simulink model "Control_Of_SinglePhaseACMotor"  (R2024b)
settings: Solver=FixedStepDiscrete  StartTime=0.0  StopTime=10.0  FixedStep=50e-6  RelTol=1e-3
undefined symbols (not defined in the file): DiscIntNeverNeededParam, Frequency
libraries: simulink x1
settings Model: DataDictionary=Control_Of_SinglePhaseACMotor.sldd  Creator=User  LastModifiedBy=User

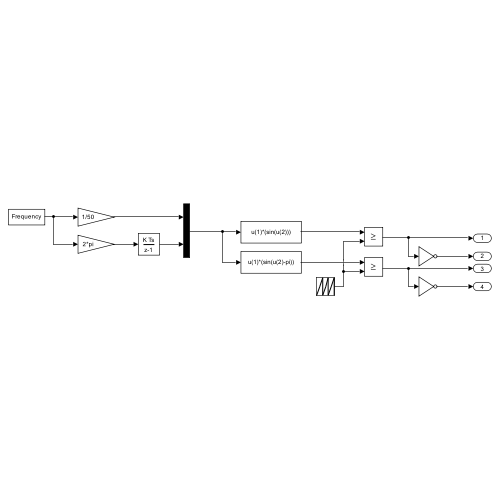
[thumbnail: Simulink's stored preview of the top-level diagram]
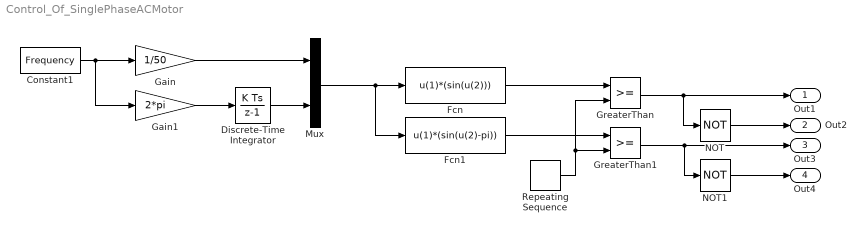
== system Control_Of_SinglePhaseACMotor ==
  Constant1 : Constant  Value=Frequency
  Discrete-Time Integrator : DiscreteIntegrator  SampleTime=-1  ICPrevOutput=DiscIntNeverNeededParam  ICPrevScaledInput=DiscIntNeverNeededParam
  Fcn : Fcn  Expr=u(1)*(sin(u(2)))
  Fcn1 : Fcn  Expr=u(1)*(sin(u(2)-pi))
  Gain : Gain  Gain=1/50
  Gain1 : Gain  Gain=2*pi
  GreaterThan : RelationalOperator  OutDataTypeStr=boolean  RndMeth=Simplest  InputSameDT=off
  GreaterThan1 : RelationalOperator  OutDataTypeStr=boolean  RndMeth=Simplest  InputSameDT=off
  Mux : Mux  Inputs=2
  NOT : Logic  Operator=NOT  IconShape=distinctive  AllPortsSameDT=off  OutDataTypeStr=boolean
  NOT1 : Logic  Operator=NOT  IconShape=distinctive  AllPortsSameDT=off  OutDataTypeStr=boolean
  Repeating Sequence : simulink/Sources/Repeating Sequence  rep_seq_t=[0 1 2]  rep_seq_y=[-1 0 1]
  Out1 : Outport
  Out2 : Outport  Port=2
  Out3 : Outport  Port=3
  Out4 : Outport  Port=4
  wires:
  Constant1/1 -> Gain1/1, Gain/1
  Gain1/1 -> Discrete-Time Integrator/1
  Gain/1 -> Mux/1
  Discrete-Time Integrator/1 -> Mux/2
  Mux/1 -> Fcn1/1, Fcn/1
  NOT1/1 -> Out4/1
  GreaterThan1/1 -> NOT1/1, Out3/1
  Repeating Sequence/1 -> GreaterThan1/2, GreaterThan/2
  Fcn1/1 -> GreaterThan1/1
  Fcn/1 -> GreaterThan/1
  GreaterThan/1 -> NOT/1, Out1/1
  NOT/1 -> Out2/1
